simulink model "desing2"  (R2024a)
settings: Solver=VariableStepAuto  StartTime=0.0  StopTime=10.0  RelTol=1e-3
undefined symbols (not defined in the file or in its folder): D1, lagging, pulse
libraries: spsThyristorLib x6, spsThreePhaseParallelRLCBranchLib x4, spsThreePhaseVIMeasurementLib x3, spsGroundLib x2, spsThreePhaseBreakerLib x2, spsPLL3phLib x1, spsPulseGeneratorThyristor6PulseLib x1, simulink x1, spsAlphaBetaZerotodq0Lib x1, slpidlib x1, spsabctoAlphaBetaZeroLib x1, spsThreePhaseProgrammableVoltageSourceLib x1
settings Model: Creator=gshma  LastModifiedBy=gshma

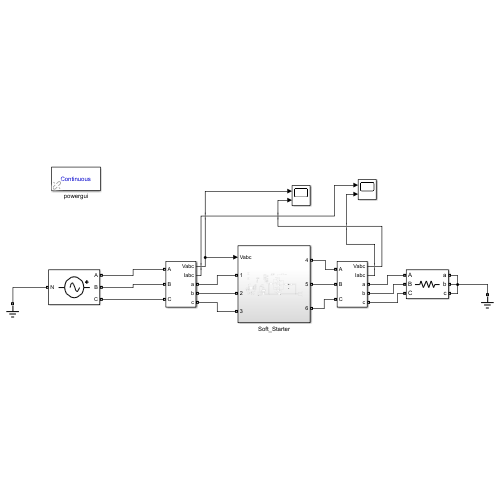
[thumbnail: Simulink's stored preview of the top-level diagram]
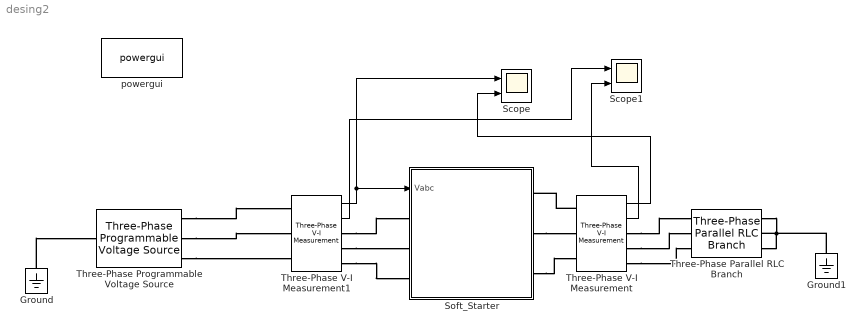
== system desing2 ==
  Ground : spsGroundLib/Ground  LConnTagsString=a
  Ground1 : spsGroundLib/Ground  LConnTagsString=a
  Scope : Scope  NumInputPorts=2
  Scope1 : Scope  NumInputPorts=2
  Soft_Starter : Subsystem
  Three-Phase Parallel RLC Branch : spsThreePhaseParallelRLCBranchLib/Three-Phase Parallel RLC Branch  LConnTagsString=A|B|C  RConnTagsString=A|B|C  BranchType=R  Resistance=10  Inductance=1e-3  Capacitance=1e-6  Measurements=None
  Three-Phase Programmable Voltage Source : spsThreePhaseProgrammableVoltageSourceLib/Three-Phase Programmable Voltage Source  PositiveSequence="[400/sqrt(2)  -30 50]"  VariationEntity=None  VariationType=Table of time-amplitude pairs  VariationTypeAlt=Step  VariationStep=0.5  VariationRate=10  VariationMagnitude=0.3  VariationFrequency=2  VariationTiming=[1 2]  VariationPhaseA=off  Amplitudes=[1 0.8 1.2 1.0]  TimeValues=[0 0.1 0.15 0.2]  HarmonicGeneration=off  HarmonicA=[3 0.2 -25 0]  HarmonicB=[2 0.15 35 2]  Timing="[0.05  3]"  BusType=swing  Pref=0  Qref=0  Qmin=-inf  Qmax=inf
  Three-Phase V-I Measurement : spsThreePhaseVIMeasurementLib/Three-Phase V-I Measurement  VoltageMeasurement=phase-to-phase  SetLabelV=off  LabelV=Vabc  Vpu=off  VpuLL=off  CurrentMeasurement=yes  SetLabelI=off  LabelI=Iabc  Ipu=off  Pbase=100e6  Vbase=500e3  OutputType=Complex  PhasorSimulation=off  PSBequivalent=0
  Three-Phase V-I Measurement1 : spsThreePhaseVIMeasurementLib/Three-Phase V-I Measurement  VoltageMeasurement=phase-to-phase  SetLabelV=off  LabelV=Vabc  Vpu=off  VpuLL=off  CurrentMeasurement=yes  SetLabelI=off  LabelI=Iabc  Ipu=off  Pbase=100e6  Vbase=500e3  OutputType=Complex  PhasorSimulation=off  PSBequivalent=0
  powergui : sps_lib/powergui  Priority=1  SimulationMode=Continuous  SampleTime=50e-6  frequency=60  Iterations=50  frequencyindice=50  Pbase=100e6  ErrMax=1e-4  UnitsV=kV  UnitsW=MW  buscounter=0  FunctionMessages=off  echomessages=off  EnableUseOfTLC=off  CurrentSourceSwitches=off  DisableSnubberDevices=on  DisableRonSwitches=on  DisableVfSwitches=on  DisplayEquations=off  AutomaticDiscreteSolvers=off  SolverType=Tustin/Backward Euler (TBE)  Interpol=off  ExternalGateDelay=off  methode=off  Ts=100  x0status=blocks  SPID=on  SwTol=0  HookPort=off  NonlinearTolerance=1e-4  nMaxIteration=100  ContinueOnMaxIteration=off  RestoreLinks=warning  ResistiveCurrentMeasurement=off  Frange=[0:2:500]  Ylog=off  Xlog=on  ShowGrid=off  save=off  variable=ZData  structure=0  ZoomFFT=off  StartTime=0.0  cycles=1  DisplayStyle=1  fundamental=60  FreqAxis=off  MaxFrequency=1000  frequencyindicesteady=1  RmsSteady=1  display=off
  wires:
  Three-Phase V-I Measurement/1 -> Scope/2
  Three-Phase V-I Measurement1/1 -> Soft_Starter/1(Vabc), Scope/1
  Three-Phase V-I Measurement1/2 -> Scope1/1
  Three-Phase V-I Measurement/2 -> Scope1/2
  connections:
  Three-Phase Parallel RLC Branch/RConn1 -- Ground1/LConn1 -- Three-Phase Parallel RLC Branch/RConn3 -- Three-Phase Parallel RLC Branch/RConn2
  Soft_Starter/RConn2 -- Three-Phase V-I Measurement/LConn2
  Three-Phase V-I Measurement/LConn1 -- Soft_Starter/RConn1
  Three-Phase V-I Measurement/RConn1 -- Three-Phase Parallel RLC Branch/LConn1
  Three-Phase V-I Measurement/RConn2 -- Three-Phase Parallel RLC Branch/LConn2
  Three-Phase V-I Measurement/RConn3 -- Three-Phase Parallel RLC Branch/LConn3
  Three-Phase V-I Measurement1/RConn2 -- Soft_Starter/LConn2
  Three-Phase V-I Measurement1/RConn1 -- Soft_Starter/LConn1
  Three-Phase V-I Measurement1/RConn3 -- Soft_Starter/LConn3
  Soft_Starter/RConn3 -- Three-Phase V-I Measurement/LConn3
  Three-Phase Programmable Voltage Source/RConn1 -- Three-Phase V-I Measurement1/LConn1
  Three-Phase Programmable Voltage Source/RConn2 -- Three-Phase V-I Measurement1/LConn2
  Three-Phase Programmable Voltage Source/RConn3 -- Three-Phase V-I Measurement1/LConn3
  Ground/LConn1 -- Three-Phase Programmable Voltage Source/LConn1

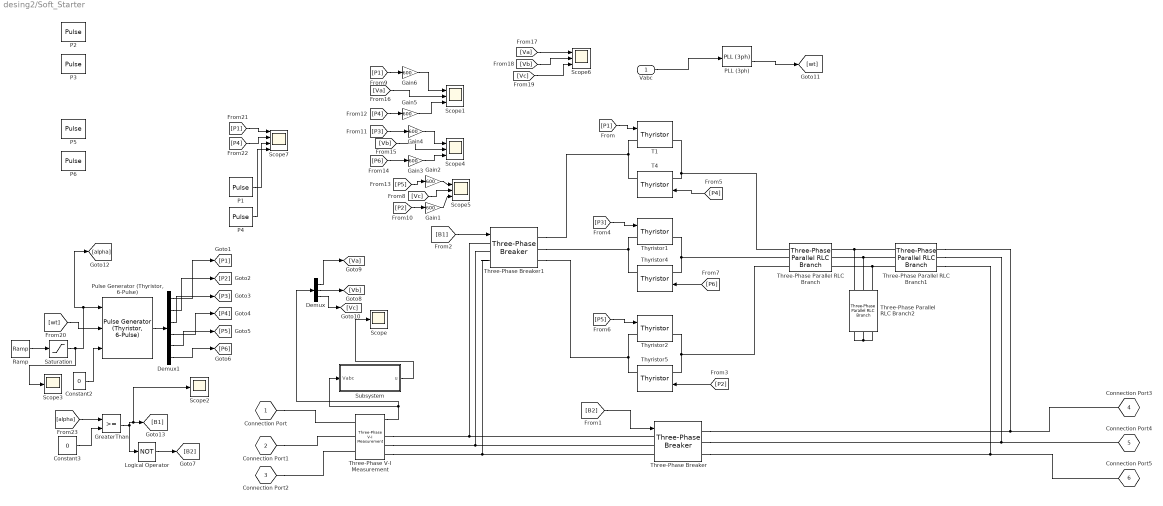
== system desing2/Soft_Starter ==
  Vabc : Inport
  Constant2 : Constant  Value=0
  Constant3 : Constant  Value=0
  Demux : Demux  Outputs=3
  Demux1 : Demux  Outputs=6
  Gain{1..6} (6 alike) : Gain  Gain=600
  GreaterThan : RelationalOperator  OutDataTypeStr=boolean  RndMeth=Simplest  InputSameDT=off
  Logical Operator : Logic  Operator=NOT  AllPortsSameDT=off  OutDataTypeStr=boolean
  "P1 " : DiscretePulseGenerator  PulseType=Time based  Period=1/50  PulseWidth=20
  P2 : DiscretePulseGenerator  PulseType=Time based  Period=1/50  PulseWidth=20  PhaseDelay=(60/360) *(1/50)
  P3 : DiscretePulseGenerator  PulseType=Time based  Period=1/50  PulseWidth=20  PhaseDelay=(120/360) *(1/50)
  P4 : DiscretePulseGenerator  PulseType=Time based  Period=1/50  PulseWidth=20  PhaseDelay=(180/360) *(1/50)
  P5 : DiscretePulseGenerator  PulseType=Time based  Period=1/50  PulseWidth=20  PhaseDelay=(240/360) *(1/50)
  P6 : DiscretePulseGenerator  PulseType=Time based  Period=1/50  PulseWidth=20  PhaseDelay=(300/360) *(1/50)
  PLL (3ph) : spsPLL3phLib/PLL (3ph)  Fmin=45  Par_Init=[0, 60]  ParK=[180, 3200, 1]  TcD=1e-4  MaxRateChangeFreq=12  FilterCutOffFreq=25  Ts=0  AGC=on
  "Pulse Generator (Thyristor, 6-Pulse)" : spsPulseGeneratorThyristor6PulseLib/Pulse Generator (Thyristor, 6-Pulse)  GenType=6-pulse  Delta=D1 (lagging)  pwidth=60  Double_Pulse=off  Ts=0
      settings: LibrarySourceBlock=|
      | sps_lib/Power Electronics/Power Electronics Control/Pulse Generator
      | (Thyristor, 6-Pulse)
  Ramp : simulink/Sources/Ramp  slope=-70  start=0.1  InitialOutput=90
  Saturation : Saturate  UpperLimit=90  LowerLimit=0
  Scope : Scope
  Scope{1,4..6} (4 alike) : Scope  NumInputPorts=3
  Scope2 : Scope
  Scope3 : Scope
  Scope7 : Scope  NumInputPorts=4
  Subsystem : Subsystem
  T1 : spsThyristorLib/Thyristor  Ron=0.001  Lon=0  Vf=0.8  IC=0  Rs=500  Cs=250e-9  Measurements=on
  T4 : spsThyristorLib/Thyristor  Ron=0.001  Lon=0  Vf=0.8  IC=0  Rs=500  Cs=250e-9  Measurements=on
  Three-Phase Parallel RLC Branch : spsThreePhaseParallelRLCBranchLib/Three-Phase Parallel RLC Branch  LConnTagsString=A|B|C  RConnTagsString=A|B|C  BranchType=L  Resistance=1  Inductance=1e-3  Capacitance=1e-6  Measurements=None
  Three-Phase Parallel RLC Branch1 : spsThreePhaseParallelRLCBranchLib/Three-Phase Parallel RLC Branch  LConnTagsString=A|B|C  RConnTagsString=A|B|C  BranchType=L  Resistance=1  Inductance=2e-3  Capacitance=1e-6  Measurements=None
  Three-Phase Parallel RLC Branch2 : spsThreePhaseParallelRLCBranchLib/Three-Phase Parallel RLC Branch  LConnTagsString=A|B|C  RConnTagsString=A|B|C  BranchType=RC  Resistance=2  Inductance=38.25e-3  Capacitance=10e-6  Measurements=None
  Three-Phase V-I Measurement : spsThreePhaseVIMeasurementLib/Three-Phase V-I Measurement  VoltageMeasurement=phase-to-phase  SetLabelV=off  LabelV=Vabc  Vpu=off  VpuLL=off  CurrentMeasurement=yes  SetLabelI=off  LabelI=Iabc  Ipu=off  Pbase=100e6  Vbase=500e3  OutputType=Complex  PhasorSimulation=off  PSBequivalent=0
  Three-Phase Breaker : spsThreePhaseBreakerLib/Three-Phase Breaker  InitialState=open  SwitchA=on  SwitchB=on  SwitchC=on  SwitchTimes="[1/60  5/60]"  External=on  BreakerResistance=0.01  SnubberResistance=1e6  SnubberCapacitance=inf  Measurements=None
  Three-Phase Breaker1 : spsThreePhaseBreakerLib/Three-Phase Breaker  InitialState=closed  SwitchA=on  SwitchB=on  SwitchC=on  SwitchTimes="[1/60  5/60]"  External=on  BreakerResistance=0.01  SnubberResistance=1e6  SnubberCapacitance=inf  Measurements=None
  Thyristor{1..2,4..5} (4 alike) : spsThyristorLib/Thyristor  Ron=0.001  Lon=0  Vf=0.8  IC=0  Rs=500  Cs=250e-9  Measurements=on
  Connection Port : PMIOPort  Tag=simrfV2util1/Connection Port  Side=Left
  Connection Port1 : PMIOPort  Tag=simrfV2util1/Connection Port  Port=2  Side=Left
  Connection Port2 : PMIOPort  Tag=simrfV2util1/Connection Port  Port=3  Side=Left
  Connection Port3 : PMIOPort  Tag=simrfV2util1/Connection Port  Port=4  Side=Right
  Connection Port4 : PMIOPort  Tag=simrfV2util1/Connection Port  Port=5  Side=Right
  Connection Port5 : PMIOPort  Tag=simrfV2util1/Connection Port  Port=6  Side=Right
  wires:
  [B2] -> Three-Phase Breaker/1
  Three-Phase V-I Measurement/1 -> Demux/1, Subsystem/1(Vabc)
  Subsystem/1(u) -> Scope/1
  [B1] -> Three-Phase Breaker1/1
  [P1] -> T1/1
  [P2] -> Thyristor5/1
  [P3] -> Thyristor1/1
  [P4] -> T4/1
  [P5] -> Thyristor2/1
  [P6] -> Thyristor4/1
  Vabc/1 -> PLL (3ph)/1
  PLL (3ph)/2 -> [wt]
  Demux/2 -> [Vb]
  Demux/1 -> [Va]
  Demux/3 -> [Vc]
  [Vc] -> Scope5/2
  [P2] -> Gain1/1
  Gain1/1 -> Scope5/3
  [P5] -> Gain2/1
  Gain2/1 -> Scope5/1
  [P6] -> Gain3/1
  Gain3/1 -> Scope4/3
  [P3] -> Gain4/1
  Gain4/1 -> Scope4/1
  [P4] -> Gain5/1
  Gain5/1 -> Scope1/3
  [P1] -> Gain6/1
  Gain6/1 -> Scope1/1
  [Vb] -> Scope4/2
  [Va] -> Scope1/2
  [Va] -> Scope6/1
  [Vb] -> Scope6/2
  [Vc] -> Scope6/3
  [wt] -> "Pulse Generator (Thyristor, 6-Pulse)"/2
  Ramp/1 -> Saturation/1
  Saturation/1 -> Scope3/1, "Pulse Generator (Thyristor, 6-Pulse)"/1, [alpha]
  Constant2/1 -> "Pulse Generator (Thyristor, 6-Pulse)"/3
  "Pulse Generator (Thyristor, 6-Pulse)"/1 -> Demux1/1
  Demux1/1 -> [P1]
  Demux1/2 -> [P2]
  Demux1/3 -> [P3]
  Demux1/4 -> [P4]
  Demux1/5 -> [P5]
  Demux1/6 -> [P6]
  [P1] -> Scope7/1
  [P4] -> Scope7/2
  "P1 "/1 -> Scope7/3
  P4/1 -> Scope7/4
  [alpha] -> GreaterThan/1
  Constant3/1 -> GreaterThan/2
  GreaterThan/1 -> Scope2/1, [B1], Logical Operator/1
  Logical Operator/1 -> [B2]
  connections:
  Three-Phase V-I Measurement/RConn2 -- Three-Phase Breaker1/LConn2 -- Three-Phase Breaker/LConn2
  Three-Phase V-I Measurement/RConn1 -- Three-Phase Breaker1/LConn1 -- Three-Phase Breaker/LConn1
  Three-Phase Breaker/RConn3 -- Three-Phase Parallel RLC Branch1/RConn3 -- Connection Port5/RConn1
  Three-Phase V-I Measurement/RConn3 -- Three-Phase Breaker1/LConn3 -- Three-Phase Breaker/LConn3
  Three-Phase Breaker/RConn1 -- Three-Phase Parallel RLC Branch1/RConn1 -- Connection Port3/RConn1
  Three-Phase Breaker/RConn2 -- Three-Phase Parallel RLC Branch1/RConn2 -- Connection Port4/RConn1
  Connection Port/RConn1 -- Three-Phase V-I Measurement/LConn1
  Connection Port1/RConn1 -- Three-Phase V-I Measurement/LConn2
  Connection Port2/RConn1 -- Three-Phase V-I Measurement/LConn3
  T4/RConn1 -- Three-Phase Breaker1/RConn1 -- T1/LConn1
  Thyristor1/LConn1 -- Thyristor4/RConn1 -- Three-Phase Breaker1/RConn2
  Thyristor2/LConn1 -- Three-Phase Breaker1/RConn3 -- Thyristor5/RConn1
  Thyristor2/RConn1 -- Three-Phase Parallel RLC Branch/LConn3 -- Thyristor5/LConn1
  T4/LConn1 -- Three-Phase Parallel RLC Branch/LConn1 -- T1/RConn1
  Thyristor1/RConn1 -- Three-Phase Parallel RLC Branch/LConn2 -- Thyristor4/LConn1
  Three-Phase Parallel RLC Branch1/LConn1 -- Three-Phase Parallel RLC Branch2/RConn1 -- Three-Phase Parallel RLC Branch/RConn1
  Three-Phase Parallel RLC Branch1/LConn2 -- Three-Phase Parallel RLC Branch2/RConn2 -- Three-Phase Parallel RLC Branch/RConn2
  Three-Phase Parallel RLC Branch1/LConn3 -- Three-Phase Parallel RLC Branch2/RConn3 -- Three-Phase Parallel RLC Branch/RConn3
  Three-Phase Parallel RLC Branch2/LConn1 -- Three-Phase Parallel RLC Branch2/LConn2 -- Three-Phase Parallel RLC Branch2/LConn3

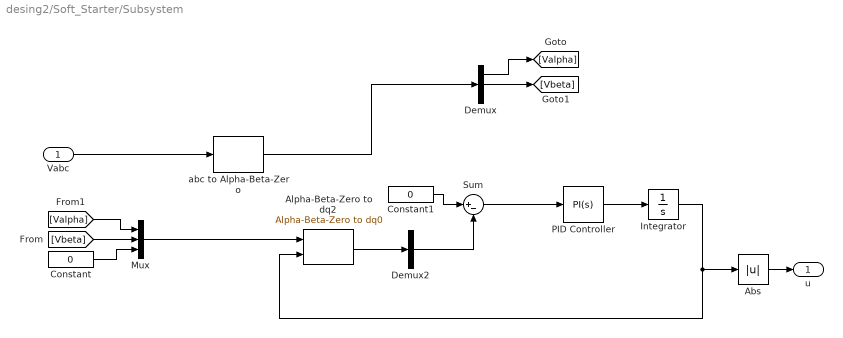
== system desing2/Soft_Starter/Subsystem ==
  Vabc : Inport
  Abs : Abs  SaturateOnIntegerOverflow=off
  Alpha-Beta-Zero to dq2 : spsAlphaBetaZerotodq0Lib/Alpha-Beta-Zero to dq0  Alignment=90 degrees behind phase A axis
  Constant : Constant  Value=0  SampleTime=0.000001
  Constant1 : Constant  Value=0  SampleTime=0.000001
  Demux : Demux  Outputs=3
  Demux2 : Demux  Outputs=3
  Integrator : Integrator
  Mux : Mux  Inputs=3
  PID Controller : slpidlib/PID Controller  Controller=PI  Form=Parallel  TimeDomain=Continuous-time  UseExternalTs=off  SampleTime=-1  IntegratorMethod=Forward Euler  FilterMethod=Forward Euler  ControllerParametersSource=internal  P=10  I=50000  UseKiTs=off  D=0  UseExternalDerivativeSource=off  N=100  UseFilter=on  TunerSelectOption=Transfer Function Based (PID Tuner App)  InitialConditionSource=internal  InitialConditionForIntegrator=0  InitialConditionForFilter=0  DifferentiatorICPrevScaledInput=0  ExternalReset=none  TrackingMode=off  Kt=1  LimitOutput=off  SatLimitsSource=internal  UpperSaturationLimit=inf  LowerSaturationLimit=-inf  LinearizeAsGain=on  AntiWindupMode=none  Kb=1  LimitIntegrator=off  UpperIntegratorSaturationLimit=inf  LowerIntegratorSaturationLimit=-inf  POutMin=[]  POutMax=[]  IOutMin=[]  IOutMax=[]  DOutMin=[]  DOutMax=[]  NOutMin=[]  NOutMax=[]  SumOutMin=[]  SumOutMax=[]  SaturationOutMin=[]  SaturationOutMax=[]  PParamMin=[]  PParamMax=[]  IParamMin=[]  IParamMax=[]  DParamMin=[]  DParamMax=[]  NParamMin=[]  NParamMax=[]  KbParamMin=[]  KbParamMax=[]  KtParamMin=[]  KtParamMax=[]  KbOutMin=[]  KbOutMax=[]  KtOutMin=[]  KtOutMax=[]  IntegratorOutMin=[]  IntegratorOutMax=[]  FilterOutMin=[]  FilterOutMax=[]  SumI1OutMin=[]  SumI1OutMax=[]  SumI2OutMin=[]  SumI2OutMax=[]  SumI3OutMin=[]  SumI3OutMax=[]  SumI4OutMin=[]  SumI4OutMax=[]  SumDOutMin=[]  SumDOutMax=[]  DifferentiatorOutMin=[]  DifferentiatorOutMax=[]  FilterDiffOutCoefMin=[]  FilterDiffOutCoefMax=[]  ReciprocalOutMin=[]  ReciprocalOutMax=[]  SumDenOutMin=[]  SumDenOutMax=[]  SumNumOutMin=[]  SumNumOutMax=[]  DivideOutMin=[]  DivideOutMax=[]  UdiffTsProdOutMin=[]  UdiffTsProdOutMax=[]  NTsProdOutMin=[]  NTsProdOutMax=[]  UintegralTsProdOutMin=[]  UintegralTsProdOutMax=[]  UngainTsProdOutMin=[]  UngainTsProdOutMax=[]  ClampingZeroOutDataTypeStr=Inherit: Inherit via back propagation  ClampingZeroOutMin=[]  ClampingZeroOutMax=[]  FilterDenConstantOutDataTypeStr=Inherit: Inherit via back propagation  FilterDenConstantOutMin=[]  FilterDenConstantOutMax=[]  PCopyOutDataTypeStr=Inherit: Inherit via back propagation  PCopyOutMin=[]  PCopyOutMax=[]  NCopyOutDataTypeStr=Inherit: Inherit via back propagation  NCopyOutMin=[]  NCopyOutMax=[]  IntegratorContinuousStateAttributes=''  IntegratorStateMustResolveToSignalObject=off  IntegratorRTWStateStorageClass=Auto  FilterContinuousStateAttributes=''  FilterStateMustResolveToSignalObject=off  FilterRTWStateStorageClass=Auto  ParallelPVariant=InternalParameters  IdealPVariant=Disabled  IVariant=InternalParameters  DVariant=Disabled  IntegratorVariant=Continuous  SatVariant=Disabled  AWVariant=Passthrough  PCopyVariant=Disabled  TRVariant=Disabled  FdbkBlocksVariant=Forward  IdealPFdbkVariant=Disabled  SatFdbkVariant=Disabled  DerivativeFilterVariant=Disabled  NVariant=Disabled  NCopyVariant=Disabled_SignalSpec  FilterICVariant=Disabled  IntegratorICVariant=InternalICs  ExternalResetVariant=Disabled  TRSumVariant=Passthrough  SumFdbkVariant=Disabled  SumVariant=Sum_PI  TsampFilterVariant=InternalTs  TsampNgainVariant=Passthrough  TsampIntegralVariant=Disabled_SignalSpec  ExternalSaturationOutDataTypeStr=Inherit: Same as second input  DerivativeSourceVariant=Disabled
  Sum : Sum  Inputs=|+-
  abc to Alpha-Beta-Zero : spsabctoAlphaBetaZeroLib/abc to Alpha-Beta-Zero
  u : Outport
  wires:
  Vabc/1 -> abc to Alpha-Beta-Zero/1
  abc to Alpha-Beta-Zero/1 -> Demux/1
  Demux/1 -> [Valpha]
  Demux/2 -> [Vbeta]
  [Vbeta] -> Mux/2
  Constant/1 -> Mux/3
  Mux/1 -> Alpha-Beta-Zero to dq2/1
  [Valpha] -> Mux/1
  Demux2/2 -> Sum/2
  Alpha-Beta-Zero to dq2/1 -> Demux2/1
  Constant1/1 -> Sum/1
  Sum/1 -> PID Controller/1
  PID Controller/1 -> Integrator/1
  Abs/1 -> u/1
  Integrator/1 -> Abs/1, Alpha-Beta-Zero to dq2/2
